simulink model "AC_AttitudeControl_sim"  (R2018b)
settings: Solver=VariableStepAuto  StartTime=0.0  StopTime=10.0  RelTol=1e-3
undefined symbols (not defined in the file or in its folder): accel_roll_max, ang_vel_pitch_max, ang_vel_roll_max, ang_vel_yaw_max, dt, HD, input_tc, rate_bf_ff_enabled
libraries: aerolibutil x7, sharedtransform x6, shared6dofsys x1
settings Model: Creator=a4327  LastModifiedBy=a4327

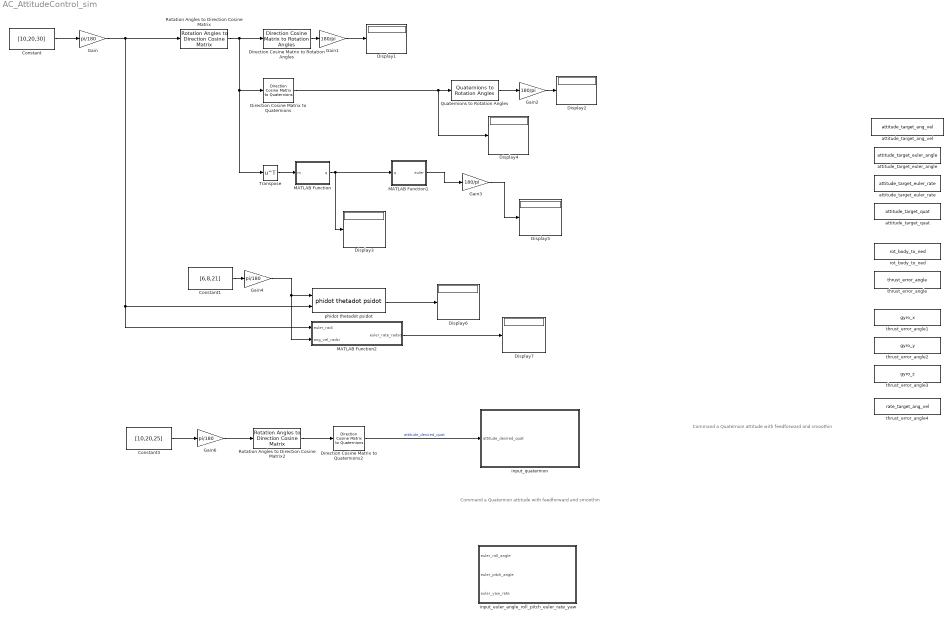
== system AC_AttitudeControl_sim ==
  note: Command a Quaternion attitude with feedforward and smoothin
  note: Command a Quaternion attitude with feedforward and smoothin
  Constant : Constant  Value=[10,20,30]
  Constant1 : Constant  Value=[6,8,21]
  Constant3 : Constant  Value=[10,20,25]
  Direction Cosine Matrix to Rotation Angles : sharedtransform/Direction Cosine Matrix to Rotation Angles  rotationOrder=ZYX  aMode=aMode  action=None  tolerance=eps(2)
      settings: SourceProductName=Aerospace Blockset  SourceProductBaseCode=AE
  Direction Cosine Matrix to Quaternions : sharedtransform/Direction Cosine Matrix  to Quaternions  aMode=0  action=None  tolerance=eps(2)
      settings: SourceProductName=Aerospace Blockset  SourceProductBaseCode=AE
  Direction Cosine Matrix to Quaternions2 : sharedtransform/Direction Cosine Matrix  to Quaternions  aMode=0  action=None  tolerance=eps(2)
      settings: SourceProductName=Aerospace Blockset  SourceProductBaseCode=AE
  Display{1..7} (7 alike) : Display
  Gain : Gain  Gain=pi/180
  Gain1 : Gain  Gain=180/pi
  Gain2 : Gain  Gain=180/pi
  Gain3 : Gain  Gain=180/pi
  Gain4 : Gain  Gain=pi/180
  Gain6 : Gain  Gain=pi/180
  MATLAB Function : MATLAB Function  TreatAsAtomicUnit=on
  MATLAB Function1 : MATLAB Function  TreatAsAtomicUnit=on
  MATLAB Function2 : MATLAB Function  TreatAsAtomicUnit=on
  Quaternions to Rotation Angles : sharedtransform/Quaternions to Rotation Angles  rotationOrder=ZYX  aMode=aMode
      settings: SourceProductBaseCode=AE
  Rotation Angles to Direction Cosine Matrix : sharedtransform/Rotation Angles to Direction Cosine Matrix  rotationOrder=ZYX  aMode=aMode
      settings: SourceProductBaseCode=AE
  Rotation Angles to Direction Cosine Matrix2 : sharedtransform/Rotation Angles to Direction Cosine Matrix  rotationOrder=ZYX  aMode=aMode
      settings: SourceProductBaseCode=AE
  Transpose : Math  Operator=transpose  SaturateOnIntegerOverflow=on
  attitude_target_ang_vel : DataStoreMemory  DataStoreName=attitude_target_ang_vel  ReadBeforeWriteMsg=warning  WriteAfterWriteMsg=warning  WriteAfterReadMsg=warning  InitialValue=attitude_target_ang_vel  ShowAdditionalParam=off
  attitude_target_euler_angle : DataStoreMemory  DataStoreName=attitude_target_euler_angle  ReadBeforeWriteMsg=warning  WriteAfterWriteMsg=warning  WriteAfterReadMsg=warning  InitialValue=attitude_target_euler_angle  ShowAdditionalParam=off
  attitude_target_euler_rate : DataStoreMemory  DataStoreName=attitude_target_euler_rate  ReadBeforeWriteMsg=warning  WriteAfterWriteMsg=warning  WriteAfterReadMsg=warning  InitialValue=attitude_target_euler_rate  ShowAdditionalParam=off
  attitude_target_quat : DataStoreMemory  DataStoreName=attitude_target_quat  ReadBeforeWriteMsg=warning  WriteAfterWriteMsg=warning  WriteAfterReadMsg=warning  InitialValue=attitude_target_quat  ShowAdditionalParam=off
  input_euler_angle_roll_pitch_euler_rate_yaw : Subsystem
  input_quaternion : Subsystem
  phidot thetadot psidot : shared6dofsys/DCM & Euler Angles (Euler)/phidot thetadot psidot  SystemSampleTime=-1
      settings: SourceProductName=Aerospace Blockset  SourceProductBaseCode=AE
  rot_body_to_ned : DataStoreMemory  DataStoreName=rot_body_to_ned  ReadBeforeWriteMsg=warning  WriteAfterWriteMsg=warning  WriteAfterReadMsg=warning  InitialValue=rot_body_to_ned  ShowAdditionalParam=off
  thrust_error_angle : DataStoreMemory  DataStoreName=thrust_error_angle  ReadBeforeWriteMsg=warning  WriteAfterWriteMsg=warning  WriteAfterReadMsg=warning  InitialValue=attitude_target_quat  ShowAdditionalParam=off
  thrust_error_angle1 : DataStoreMemory  DataStoreName=gyro_x  ReadBeforeWriteMsg=warning  WriteAfterWriteMsg=warning  WriteAfterReadMsg=warning  InitialValue=attitude_target_quat  ShowAdditionalParam=off
  thrust_error_angle2 : DataStoreMemory  DataStoreName=gyro_y  ReadBeforeWriteMsg=warning  WriteAfterWriteMsg=warning  WriteAfterReadMsg=warning  InitialValue=attitude_target_quat  ShowAdditionalParam=off
  thrust_error_angle3 : DataStoreMemory  DataStoreName=gyro_z  ReadBeforeWriteMsg=warning  WriteAfterWriteMsg=warning  WriteAfterReadMsg=warning  InitialValue=attitude_target_quat  ShowAdditionalParam=off
  thrust_error_angle4 : DataStoreMemory  DataStoreName=rate_target_ang_vel  ReadBeforeWriteMsg=warning  WriteAfterWriteMsg=warning  WriteAfterReadMsg=warning  InitialValue=attitude_target_quat  ShowAdditionalParam=off
  wires:
  Gain/1 -> MATLAB Function2/1(euler_radi), phidot thetadot psidot/2, Rotation Angles to Direction Cosine Matrix/1
  Constant/1 -> Gain/1
  Rotation Angles to Direction Cosine Matrix/1 -> Transpose/1, Direction Cosine Matrix to Quaternions/1, Direction Cosine Matrix to Rotation Angles/1
  Direction Cosine Matrix to Rotation Angles/1 -> Gain1/1
  Gain1/1 -> Display1/1
  Direction Cosine Matrix to Quaternions/1 -> Display4/1, Quaternions to Rotation Angles/1
  Quaternions to Rotation Angles/1 -> Gain2/1
  Gain2/1 -> Display2/1
  MATLAB Function/1(q) -> MATLAB Function1/1(q), Display3/1
  Transpose/1 -> MATLAB Function/1(m)
  MATLAB Function1/1(euler) -> Gain3/1
  Gain3/1 -> Display5/1
  Constant1/1 -> Gain4/1
  Gain4/1 -> MATLAB Function2/2(ang_vel_radsi), phidot thetadot psidot/1
  MATLAB Function2/1(euler_rate_radso) -> Display7/1
  phidot thetadot psidot/1 -> Display6/1
  Rotation Angles to Direction Cosine Matrix2/1 -> Direction Cosine Matrix to Quaternions2/1
  Constant3/1 -> Gain6/1
  Gain6/1 -> Rotation Angles to Direction Cosine Matrix2/1
  Direction Cosine Matrix to Quaternions2/1 -> input_quaternion/1(attitude_desired_quat)  "attitude_desired_quat"

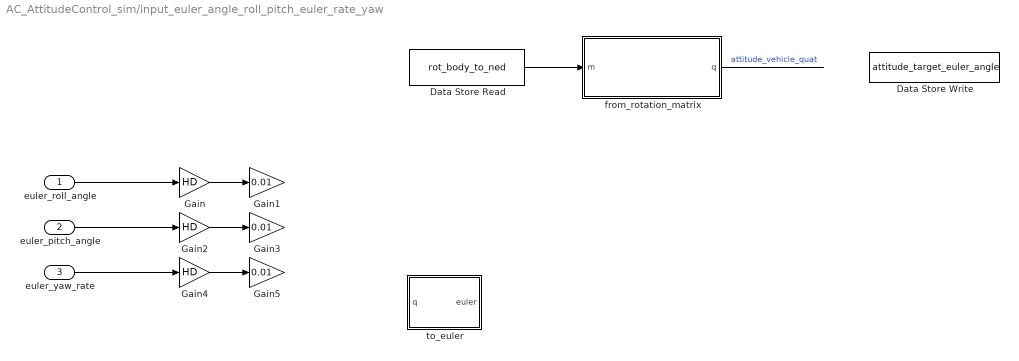
== system AC_AttitudeControl_sim/input_euler_angle_roll_pitch_euler_rate_yaw ==
  euler_roll_angle : Inport
  euler_pitch_angle : Inport  Port=2
  euler_yaw_rate : Inport  Port=3
  Data Store Read : DataStoreRead  DataStoreName=rot_body_to_ned
  Data Store Write : DataStoreWrite  DataStoreName=attitude_target_euler_angle
  Gain : Gain  Gain=HD
  Gain1 : Gain  Gain=0.01
  Gain2 : Gain  Gain=HD
  Gain3 : Gain  Gain=0.01
  Gain4 : Gain  Gain=HD
  Gain5 : Gain  Gain=0.01
  from_rotation_matrix : MATLAB Function  TreatAsAtomicUnit=on
  to_euler : MATLAB Function  TreatAsAtomicUnit=on
  wires:
  euler_roll_angle/1 -> Gain/1
  Gain/1 -> Gain1/1
  Gain2/1 -> Gain3/1
  euler_pitch_angle/1 -> Gain2/1
  Gain4/1 -> Gain5/1
  euler_yaw_rate/1 -> Gain4/1
  Data Store Read/1 -> from_rotation_matrix/1(m)
  from_rotation_matrix/1(q) -> ?  "attitude_vehicle_quat"

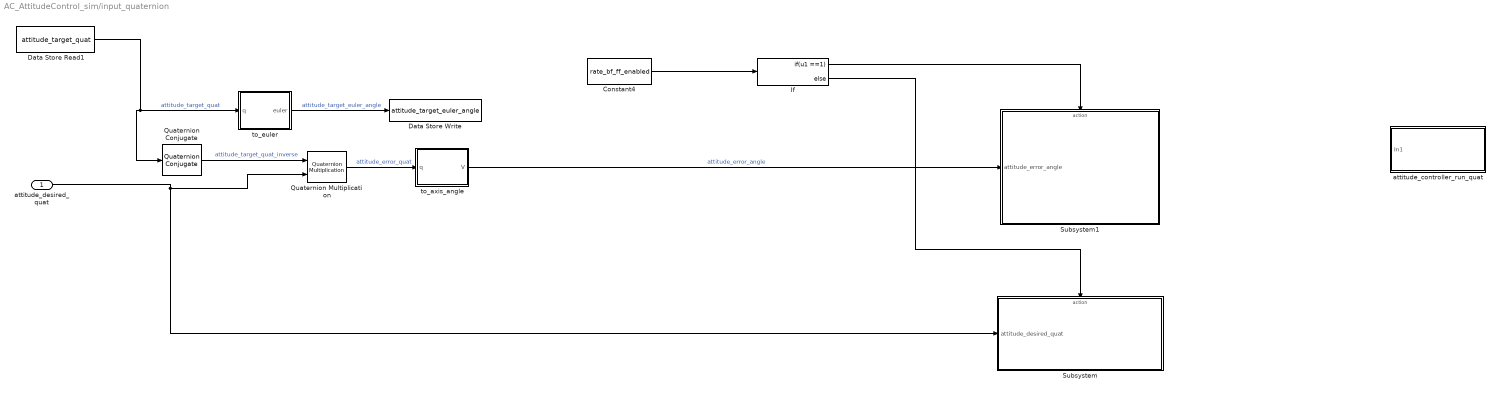
== system AC_AttitudeControl_sim/input_quaternion ==
  attitude_desired_quat : Inport
  Constant4 : Constant  Value=rate_bf_ff_enabled
  Data Store Read1 : DataStoreRead  DataStoreName=attitude_target_quat
  Data Store Write : DataStoreWrite  DataStoreName=attitude_target_euler_angle
  If : If  IfExpression=u1 ==1
  Quaternion Conjugate : aerolibutil/Quaternion Conjugate
      settings: SourceProductName=Aerospace Blockset  SourceProductBaseCode=AE
  Quaternion Multiplication : aerolibutil/Quaternion Multiplication
  Subsystem : Subsystem
  Subsystem1 : Subsystem
  attitude_controller_run_quat : Subsystem
  to_axis_angle : MATLAB Function  TreatAsAtomicUnit=on
  to_euler : MATLAB Function  TreatAsAtomicUnit=on
  wires:
  attitude_desired_quat/1 -> Subsystem/1(attitude_desired_quat), Quaternion Multiplication/2
  Quaternion Conjugate/1 -> Quaternion Multiplication/1  "attitude_target_quat_inverse"
  Data Store Read1/1 -> to_euler/1(q), Quaternion Conjugate/1  "attitude_target_quat"
  Quaternion Multiplication/1 -> to_axis_angle/1(q)  "attitude_error_quat"
  Constant4/1 -> If/1
  to_axis_angle/1(V) -> Subsystem1/1(attitude_error_angle)  "attitude_error_angle"
  If/1 -> Subsystem1/Action
  If/2 -> Subsystem/Action
  to_euler/1(euler) -> Data Store Write/1  "attitude_target_euler_angle"

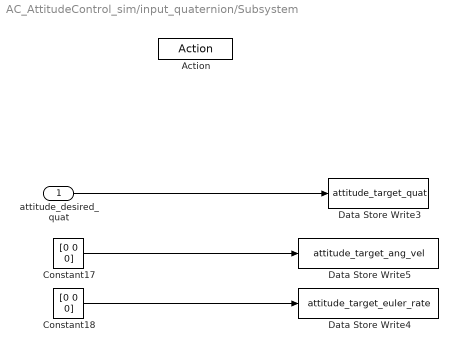
== system AC_AttitudeControl_sim/input_quaternion/Subsystem ==
  attitude_desired_quat : Inport
  Action : ActionPort  ActionType=else
  Constant17 : Constant  Value=[0 0 0]
  Constant18 : Constant  Value=[0 0 0]
  Data Store Write3 : DataStoreWrite  DataStoreName=attitude_target_quat
  Data Store Write4 : DataStoreWrite  DataStoreName=attitude_target_euler_rate
  Data Store Write5 : DataStoreWrite  DataStoreName=attitude_target_ang_vel
  wires:
  Constant18/1 -> Data Store Write4/1
  Constant17/1 -> Data Store Write5/1
  attitude_desired_quat/1 -> Data Store Write3/1

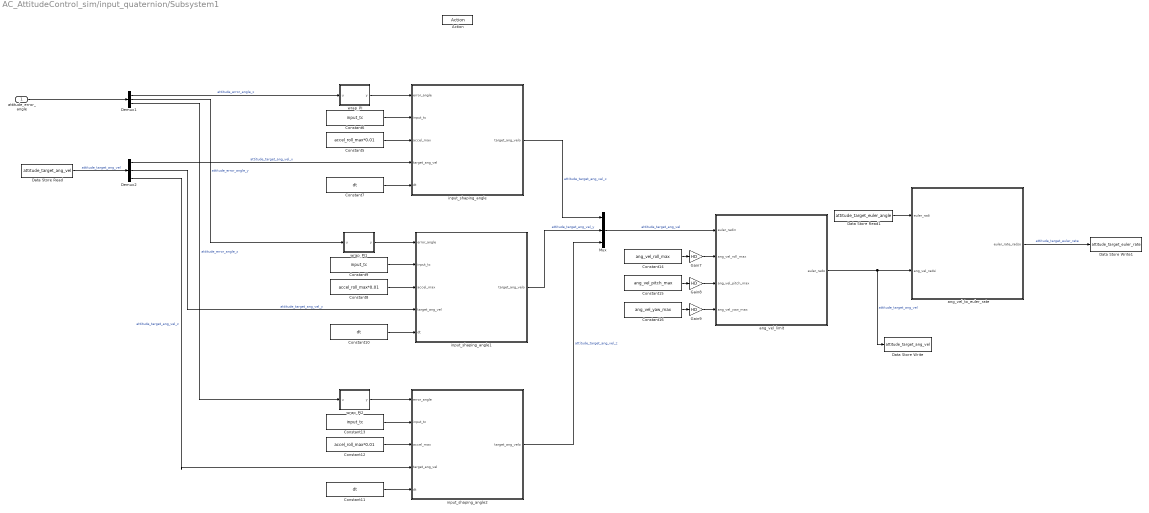
== system AC_AttitudeControl_sim/input_quaternion/Subsystem1 ==
  attitude_error_angle : Inport
  Action : ActionPort  ActionType=then
  Constant10 : Constant  Value=dt
  Constant11 : Constant  Value=dt
  Constant12 : Constant  Value=accel_roll_max*0.01
  Constant13 : Constant  Value=input_tc
  Constant14 : Constant  Value=ang_vel_roll_max
  Constant15 : Constant  Value=ang_vel_pitch_max
  Constant16 : Constant  Value=ang_vel_yaw_max
  Constant5 : Constant  Value=accel_roll_max*0.01
  Constant6 : Constant  Value=input_tc
  Constant7 : Constant  Value=dt
  Constant8 : Constant  Value=accel_roll_max*0.01
  Constant9 : Constant  Value=input_tc
  Data Store Read : DataStoreRead  DataStoreName=attitude_target_ang_vel
  Data Store Read1 : DataStoreRead  DataStoreName=attitude_target_euler_angle
  Data Store Write : DataStoreWrite  DataStoreName=attitude_target_ang_vel
  Data Store Write1 : DataStoreWrite  DataStoreName=attitude_target_euler_rate
  Demux1 : Demux  Outputs=3
  Demux2 : Demux  Outputs=3
  Gain7 : Gain  Gain=HD
  Gain8 : Gain  Gain=HD
  Gain9 : Gain  Gain=HD
  Mux : Mux  Inputs=3
  ang_vel_limit : MATLAB Function  TreatAsAtomicUnit=on
  ang_vel_to_euler_rate : MATLAB Function  TreatAsAtomicUnit=on
  input_shaping_angle : MATLAB Function  TreatAsAtomicUnit=on
  input_shaping_angle1 : MATLAB Function  TreatAsAtomicUnit=on
  input_shaping_angle2 : MATLAB Function  TreatAsAtomicUnit=on
  wrap_PI : MATLAB Function  TreatAsAtomicUnit=on
  wrap_PI1 : MATLAB Function  TreatAsAtomicUnit=on
  wrap_PI2 : MATLAB Function  TreatAsAtomicUnit=on
  wires:
  Gain9/1 -> ang_vel_limit/4(ang_vel_yaw_max)
  Gain7/1 -> ang_vel_limit/2(ang_vel_roll_max)
  input_shaping_angle/1(target_ang_velo) -> Mux/1  "attitude_target_ang_vel_x"
  Demux1/3 -> wrap_PI2/1(u)  "attitude_error_angle_z"
  ang_vel_limit/1(euler_rado) -> ang_vel_to_euler_rate/2(ang_vel_radsi), Data Store Write/1  "attitude_target_ang_vel"
  Demux1/1 -> wrap_PI/1(u)  "attitude_error_angle_x"
  input_shaping_angle1/1(target_ang_velo) -> Mux/2  "attitude_target_ang_vel_y"
  Constant12/1 -> input_shaping_angle2/3(accel_max)
  Demux2/3 -> input_shaping_angle2/4(target_ang_vel)  "attitude_target_ang_vel_z"
  Constant9/1 -> input_shaping_angle1/2(input_tc)
  input_shaping_angle2/1(target_ang_velo) -> Mux/3  "attitude_target_ang_vel_z"
  Constant5/1 -> input_shaping_angle/3(accel_max)
  Constant8/1 -> input_shaping_angle1/3(accel_max)
  Constant10/1 -> input_shaping_angle1/5(dt)
  Gain8/1 -> ang_vel_limit/3(ang_vel_pitch_max)
  Constant14/1 -> Gain7/1
  wrap_PI1/1(y) -> input_shaping_angle1/1(error_angle)
  Demux2/1 -> input_shaping_angle/4(target_ang_vel)  "attitude_target_ang_vel_x"
  wrap_PI2/1(y) -> input_shaping_angle2/1(error_angle)
  Constant7/1 -> input_shaping_angle/5(dt)
  wrap_PI/1(y) -> input_shaping_angle/1(error_angle)
  Constant11/1 -> input_shaping_angle2/5(dt)
  Demux1/2 -> wrap_PI1/1(u)  "attitude_error_angle_y"
  Constant13/1 -> input_shaping_angle2/2(input_tc)
  Constant15/1 -> Gain8/1
  Constant6/1 -> input_shaping_angle/2(input_tc)
  Data Store Read1/1 -> ang_vel_to_euler_rate/1(euler_radi)
  Constant16/1 -> Gain9/1
  Mux/1 -> ang_vel_limit/1(euler_radin)  "attitude_target_ang_vel"
  Demux2/2 -> input_shaping_angle1/4(target_ang_vel)  "attitude_target_ang_vel_y"
  ang_vel_to_euler_rate/1(euler_rate_radso) -> Data Store Write1/1  "attitude_target_euler_rate"
  Data Store Read/1 -> Demux2/1  "attitude_target_ang_vel"
  attitude_error_angle/1 -> Demux1/1

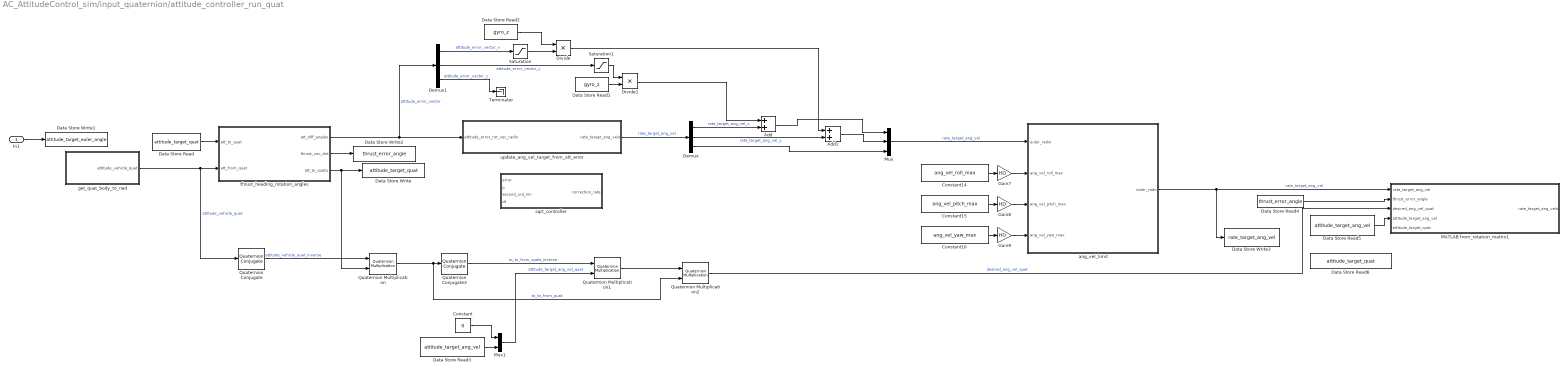
== system AC_AttitudeControl_sim/input_quaternion/attitude_controller_run_quat ==
  In1 : Inport
  Add : Sum
  Add1 : Sum
  Constant : Constant  Value=0
  Constant14 : Constant  Value=ang_vel_roll_max
  Constant15 : Constant  Value=ang_vel_pitch_max
  Constant16 : Constant  Value=ang_vel_yaw_max
  Data Store Read : DataStoreRead  DataStoreName=attitude_target_quat
  Data Store Read1 : DataStoreRead  DataStoreName=gyro_z
  Data Store Read2 : DataStoreRead  DataStoreName=gyro_z
  Data Store Read3 : DataStoreRead  DataStoreName=attitude_target_ang_vel
  Data Store Read4 : DataStoreRead  DataStoreName=thrust_error_angle
  Data Store Read5 : DataStoreRead  DataStoreName=attitude_target_ang_vel
  Data Store Read6 : DataStoreRead  DataStoreName=attitude_target_quat
  Data Store Write : DataStoreWrite  DataStoreName=attitude_target_quat
  Data Store Write1 : DataStoreWrite  DataStoreName=attitude_target_euler_angle
  Data Store Write2 : DataStoreWrite  DataStoreName=thrust_error_angle
  Data Store Write3 : DataStoreWrite  DataStoreName=rate_target_ang_vel
  Demux : Demux  Outputs=3
  Demux1 : Demux  Outputs=3
  Divide : Product  Inputs=**
  Divide1 : Product  Inputs=**
  Gain7 : Gain  Gain=HD
  Gain8 : Gain  Gain=HD
  Gain9 : Gain  Gain=HD
  MATLAB from_rotation_matrix1 : MATLAB Function  TreatAsAtomicUnit=on
  Mux : Mux  Inputs=3
  Mux1 : Mux  Inputs=2
  Quaternion Conjugate : aerolibutil/Quaternion Conjugate
      settings: SourceProductName=Aerospace Blockset  SourceProductBaseCode=AE
  Quaternion Conjugate3 : aerolibutil/Quaternion Conjugate
      settings: SourceProductName=Aerospace Blockset  SourceProductBaseCode=AE
  Quaternion Multiplication : aerolibutil/Quaternion Multiplication
  Quaternion Multiplication1 : aerolibutil/Quaternion Multiplication
  Quaternion Multiplication2 : aerolibutil/Quaternion Multiplication
  Saturation : Saturate  UpperLimit=pi/4  LowerLimit=-pi/4
  Saturation1 : Saturate  UpperLimit=pi/4  LowerLimit=-pi/4
  Terminator : Terminator
  ang_vel_limit : MATLAB Function  TreatAsAtomicUnit=on
  get_quat_body_to_ned : Subsystem
  sqrt_controller : MATLAB Function  TreatAsAtomicUnit=on
  thrust_heading_rotation_angles : MATLAB Function  TreatAsAtomicUnit=on
  update_ang_vel_target_from_att_error : MATLAB Function  TreatAsAtomicUnit=on
  wires:
  In1/1 -> Data Store Write1/1
  Data Store Read/1 -> thrust_heading_rotation_angles/1(att_to_quat)
  get_quat_body_to_ned/1(attitude_vehicle_quat) -> Quaternion Conjugate/1, thrust_heading_rotation_angles/2(att_from_quat)  "attitude_vehicle_quat"
  thrust_heading_rotation_angles/1(att_diff_angleo) -> Demux1/1, update_ang_vel_target_from_att_error/1(attitude_error_rot_vec_radin)  "attitude_error_vector"
  thrust_heading_rotation_angles/2(thrust_vec_dot) -> Data Store Write2/1
  update_ang_vel_target_from_att_error/1(rate_target_ang_velo) -> Demux/1  "rate_target_ang_vel"
  Demux1/2 -> Saturation1/1  "attitude_error_vector_y"
  Demux1/1 -> Saturation/1  "attitude_error_vector_x"
  Demux1/3 -> Terminator/1  "attitude_error_vector_z"
  Saturation/1 -> Divide/2
  Data Store Read2/1 -> Divide/1
  Saturation1/1 -> Divide1/1
  Data Store Read1/1 -> Divide1/2
  Demux/2 -> Add1/2  "rate_target_ang_vel_y"
  Demux/1 -> Add/2  "rate_target_ang_vel_x"
  Divide1/1 -> Add/1
  Divide/1 -> Add1/1
  Demux/3 -> Mux/3
  Add/1 -> Mux/1
  Add1/1 -> Mux/2
  Mux/1 -> ang_vel_limit/1(euler_radin)  "rate_target_ang_vel"
  Constant16/1 -> Gain9/1
  Constant15/1 -> Gain8/1
  Gain8/1 -> ang_vel_limit/3(ang_vel_pitch_max)
  Gain7/1 -> ang_vel_limit/2(ang_vel_roll_max)
  ang_vel_limit/1(euler_rado) -> MATLAB from_rotation_matrix1/1(rate_target_ang_vel), Data Store Write3/1  "rate_target_ang_vel"
  Constant14/1 -> Gain7/1
  Gain9/1 -> ang_vel_limit/4(ang_vel_yaw_max)
  Data Store Read3/1 -> Mux1/2
  Constant/1 -> Mux1/1
  Quaternion Conjugate/1 -> Quaternion Multiplication/1  "attitude_vehicle_quat_inverse"
  thrust_heading_rotation_angles/3(att_to_quato) -> Quaternion Multiplication/2, Data Store Write/1
  Quaternion Multiplication/1 -> Quaternion Multiplication2/2, Quaternion Conjugate3/1  "to_to_from_quat"
  Quaternion Conjugate3/1 -> Quaternion Multiplication1/1  "to_to_from_quatt_inverse"
  Mux1/1 -> Quaternion Multiplication1/2  "attitude_target_ang_vel_quat"
  Quaternion Multiplication1/1 -> Quaternion Multiplication2/1
  Quaternion Multiplication2/1 -> MATLAB from_rotation_matrix1/3(desired_ang_vel_quat)  "desired_ang_vel_quat"
  Data Store Read4/1 -> MATLAB from_rotation_matrix1/2(thrust_error_angle)
  Data Store Read5/1 -> MATLAB from_rotation_matrix1/4(attitude_target_ang_vel)

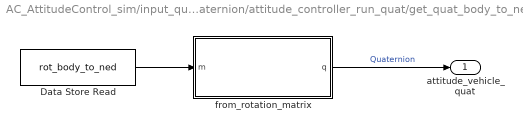
== system AC_AttitudeControl_sim/input_quaternion/attitude_controller_run_quat/get_quat_body_to_ned ==
  Data Store Read : DataStoreRead  DataStoreName=rot_body_to_ned
  from_rotation_matrix : MATLAB Function  TreatAsAtomicUnit=on
  attitude_vehicle_quat : Outport
  wires:
  from_rotation_matrix/1(q) -> attitude_vehicle_quat/1  "Quaternion"
  Data Store Read/1 -> from_rotation_matrix/1(m)

== matlab function AC_AttitudeControl_sim/MATLAB Function1 ==
  data: q input; euler output
function euler = fcn(q)
[roll, pitch, yaw]=q_to_euler(q);
euler=[yaw, pitch,roll ];
end

== matlab function AC_AttitudeControl_sim/MATLAB Function ==
  data: m input; q output
function q = fcn(m)
q=from_rotation_matrix(m);
end

== matlab function AC_AttitudeControl_sim/MATLAB Function2 ==
  data: euler_radi input; euler_rate_radso output; ang_vel_radsi input
function euler_rate_radso = fcn(euler_radi,ang_vel_radsi)
euler_rate_radso = ang_vel_to_euler_rate(euler_radi,ang_vel_radsi);
end

== matlab function AC_AttitudeControl_sim/input_quaternion/to_euler ==
  data: q input; euler output
function euler = to_euler(q)
q1=q(1);
q2=q(2);
q3=q(3);
q4=q(4);
roll=atan2(2.0*(q1*q2 + q3*q4), 1.0 - 2.0*(q2*q2 + q3*q3));
pitch=asin(2.0*(q1*q3 - q4*q2));
yaw=atan2(2.0*(q1*q4 + q2*q3), 1.0 - 2.0*(q3*q3 + q4*q4));
euler=[roll, pitch, yaw];
end

== matlab function AC_AttitudeControl_sim/input_quaternion/to_axis_angle ==
  data: q input; V output
function V = to_axis_angle(q)
I=norm(q(2:4),2);
V=q(2:4);
    if(I~=0)
    V=V/I;
    V=wrap_PI(2*atan2(I,q(1)))*V;
    end 
end

== matlab function AC_AttitudeControl_sim/input_quaternion/Subsystem1/input_shaping_angle ==
  data: error_angle input; target_ang_velo output; input_tc input; accel_max input; target_ang_vel input; dt input
function target_ang_velo = input_shaping_angle(  error_angle,  input_tc,  accel_max,  target_ang_vel,  dt)
desired_ang_vel = sqrt_controller(error_angle, 1.0/ max(input_tc, 0.01), accel_max, dt);
   % Acceleration is limited directly to smooth the beginning of the curve.
     target_ang_velo=input_shaping_ang_vel(target_ang_vel, desired_ang_vel, accel_max, dt);
end

== matlab function AC_AttitudeControl_sim/input_quaternion/Subsystem1/wrap_PI ==
  data: u input; y output
function y = wrap_PI(u)
y = wrap_PI(u);

== matlab function AC_AttitudeControl_sim/input_quaternion/Subsystem1/input_shaping_angle1 ==
  data: error_angle input; target_ang_velo output; input_tc input; accel_max input; target_ang_vel input; dt input
function target_ang_velo = input_shaping_angle(  error_angle,  input_tc,  accel_max,  target_ang_vel,  dt)
desired_ang_vel = sqrt_controller(error_angle, 1.0/ max(input_tc, 0.01), accel_max, dt);
   % Acceleration is limited directly to smooth the beginning of the curve.
     target_ang_velo=input_shaping_ang_vel(target_ang_vel, desired_ang_vel, accel_max, dt);
end

== matlab function AC_AttitudeControl_sim/input_quaternion/Subsystem1/wrap_PI1 ==
  data: u input; y output
function y = wrap_PI(u)
y = wrap_PI(u);

== matlab function AC_AttitudeControl_sim/input_quaternion/Subsystem1/input_shaping_angle2 ==
  data: error_angle input; target_ang_velo output; input_tc input; accel_max input; target_ang_vel input; dt input
function target_ang_velo = input_shaping_angle(  error_angle,  input_tc,  accel_max,  target_ang_vel,  dt)
desired_ang_vel = sqrt_controller(error_angle, 1.0/ max(input_tc, 0.01), accel_max, dt);
   % Acceleration is limited directly to smooth the beginning of the curve.
     target_ang_velo=input_shaping_ang_vel(target_ang_vel, desired_ang_vel, accel_max, dt);
end

== matlab function AC_AttitudeControl_sim/input_quaternion/Subsystem1/wrap_PI2 ==
  data: u input; y output
function y = wrap_PI(u)
y = wrap_PI(u);

== matlab function AC_AttitudeControl_sim/input_quaternion/Subsystem1/ang_vel_limit ==
  data: euler_radin input; euler_rado output; ang_vel_roll_max input; ang_vel_pitch_max input; ang_vel_yaw_max input
function euler_rado = ang_vel_limit(  euler_radin, ang_vel_roll_max,  ang_vel_pitch_max,  ang_vel_yaw_max)
 euler_rado=ang_vel_limit( euler_radin, ang_vel_roll_max,  ang_vel_pitch_max,  ang_vel_yaw_max); 
end

== matlab function AC_AttitudeControl_sim/input_quaternion/Subsystem1/ang_vel_to_euler_rate ==
  data: euler_radi input; euler_rate_radso output; ang_vel_radsi input
function euler_rate_radso = ang_vel_to_euler_rate(euler_radi,ang_vel_radsi)
 euler_rate_radso = ang_vel_to_euler_rate(euler_radi,ang_vel_radsi); 
end

== matlab function AC_AttitudeControl_sim/input_euler_angle_roll_pitch_euler_rate_yaw/to_euler ==
  data: q input; euler output
function euler = to_euler(q)
q1=q(1);
q2=q(2);
q3=q(3);
q4=q(4);
roll=atan2(2.0*(q1*q2 + q3*q4), 1.0 - 2.0*(q2*q2 + q3*q3));
pitch=asin(2.0*(q1*q3 - q4*q2));
yaw=atan2(2.0*(q1*q4 + q2*q3), 1.0 - 2.0*(q3*q3 + q4*q4));
euler=[roll, pitch, yaw];
end

== matlab function AC_AttitudeControl_sim/input_quaternion/attitude_controller_run_quat/thrust_heading_rotation_angles ==
  data: att_to_quat input; att_diff_angleo output; att_from_quat input; thrust_vec_dot output; att_to_quato output
function [att_diff_angleo,thrust_vec_dot,att_to_quato]= thrust_heading_rotation_angles ( att_to_quat, att_from_quat)

[att_diff_angleo,thrust_vec_dot,att_to_quato]= thrust_heading_rotation_angles ( att_to_quat, att_from_quat);

end

== matlab function AC_AttitudeControl_sim/input_euler_angle_roll_pitch_euler_rate_yaw/from_rotation_matrix ==
  data: m input; q output
function q = from_rotation_matrix(m)
q=from_rotation_matrix(m);
end

== matlab function AC_AttitudeControl_sim/input_quaternion/attitude_controller_run_quat/get_quat_body_to_ned/from_rotation_matrix ==
  data: m input; q output
function q = from_rotation_matrix(m)
q=from_rotation_matrix(m);
end

== matlab function AC_AttitudeControl_sim/input_quaternion/attitude_controller_run_quat/MATLAB from_rotation_matrix1 ==
  data: rate_target_ang_vel input; rate_target_ang_velo output; thrust_error_angle input; desired_ang_vel_quat input; attitude_target_ang_vel input; attitude_target_quat input
function rate_target_ang_velo = attitude_controller_run_quat_sub1(rate_target_ang_vel,thrust_error_angle,desired_ang_vel_quat, attitude_target_ang_vel,attitude_target_quat)
%%%%%%%%待调试
global AC_ATTITUDE_THRUST_ERROR_ANGLE
global dt
    % Correct the thrust vector and smoothly add feedforward and yaw input
    if (thrust_error_angle > AC_ATTITUDE_THRUST_ERROR_ANGLE * 2.0) 
        rate_target_ang_vel.z = gyro_z;
    elseif (thrust_error_angle > AC_ATTITUDE_THRUST_ERROR_ANGLE) 
       feedforward_scalar = (1.0 - (thrust_error_angle - AC_ATTITUDE_THRUST_ERROR_ANGLE) / AC_ATTITUDE_THRUST_ERROR_ANGLE);
        rate_target_ang_vel.x =rate_target_ang_vel.x + desired_ang_vel_quat.q2 * feedforward_scalar;
        rate_target_ang_vel.y= rate_target_ang_vel.y + desired_ang_vel_quat.q3 * feedforward_scalar;
        rate_target_ang_vel.z =rate_target_ang_vel.z + desired_ang_vel_quat.q4;
        rate_target_ang_vel.z = gyro_z * (1.0 - feedforward_scalar) + rate_target_ang_vel.z * feedforward_scalar;
   else 
        rate_target_ang_vel.x =rate_target_ang_vel.x+ desired_ang_vel_quat.q2;
        rate_target_ang_vel.y =rate_target_ang_vel.y+ desired_ang_vel_quat.q3;
        rate_target_ang_vel.z =rate_target_ang_vel.z+ desired_ang_vel_quat.q4;
    end
    rate_target_ang_velo=[rate_target_ang_vel.x rate_target_ang_vel.y rate_target_ang_vel.z];

    if (rate_bf_ff_enabled) 
        % rotate target and normalize     
        attitude_target_update_quat=from_axis_angle3([attitude_target_ang_vel.x * dt, attitude_target_ang_vel.y * dt, attitude_target_ang_vel.z * dt]);
        attitude_target_quat = attitude_target_quat * attitude_target_update_quat;
        attitude_target_quat=normalizeq(attitude_target_quat) ;
    else
        attitude_target_quat=normalizeq(attitude_target_quat) ;
    end
        attitude_ang_error = attitude_vehicle_quat.inverse() * attitude_target_quat;

 end

== matlab function AC_AttitudeControl_sim/input_quaternion/attitude_controller_run_quat/sqrt_controller ==
  data: error input; correction_rate output; p input; second_ord_lim input; dt input
function correction_rate = sqrt_controller( error,  p,  second_ord_lim, dt)
correction_rate = sqrt_controller( error,  p,  second_ord_lim, dt);
end

== matlab function AC_AttitudeControl_sim/input_quaternion/attitude_controller_run_quat/update_ang_vel_target_from_att_error ==
  data: attitude_error_rot_vec_radin input; rate_target_ang_velo output
function  rate_target_ang_velo = update_ang_vel_target_from_att_error(attitude_error_rot_vec_radin)
rate_target_ang_velo = update_ang_vel_target_from_att_error(attitude_error_rot_vec_radin);
end

== matlab function AC_AttitudeControl_sim/input_quaternion/attitude_controller_run_quat/ang_vel_limit ==
  data: euler_radin input; euler_rado output; ang_vel_roll_max input; ang_vel_pitch_max input; ang_vel_yaw_max input
function euler_rado = ang_vel_limit(  euler_radin, ang_vel_roll_max,  ang_vel_pitch_max,  ang_vel_yaw_max)
 euler_rado=ang_vel_limit( euler_radin, ang_vel_roll_max,  ang_vel_pitch_max,  ang_vel_yaw_max); 
end
